simulink model "mod2"  (R2017a)
settings: Solver=VariableStepAuto  StartTime=0.0  StopTime=10.0  RelTol=1e-3
libraries: simulink x2
settings Model: Creator=step_oda  LastModifiedBy=step_oda

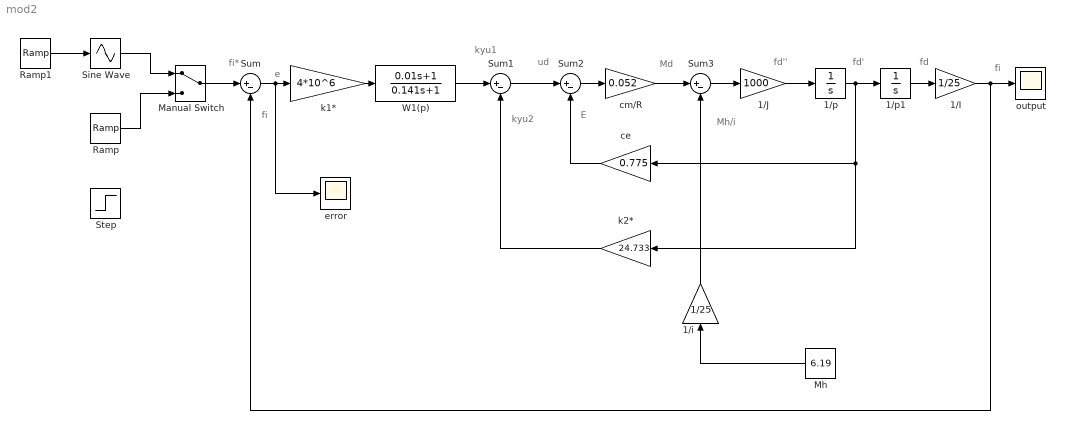
== system mod2 ==
  note: fi
  note: fd
  note: fd'
  note: fd''
  note: ud
  note: Md
  note: fi
  note: e
  note: fi*
  note: kyu1
  note: kyu2
  note: E
  note: Mh/i
  1/I : Gain  Gain=1/25
  1/J : Gain  Gain=1000
  1/i : Gain  Gain=1/25
  1/p : Integrator
  1/p1 : Integrator
  Manual Switch : ManualSwitch
  Mh : Constant  Value=6.19
  Ramp : simulink/Sources/Ramp  slope=4  start=0  X0=0
  Ramp1 : simulink/Sources/Ramp  slope=1  start=0  X0=0
  Sine Wave : Sin  TimeSource=Use external signal  Amplitude=0.533  Frequency=7.5  SampleTime=0
  Step : Step  Time=0  SampleTime=0
  Sum{,1..3} (4 alike) : Sum  Inputs=|+-
  W1(p) : TransferFcn  Numerator=[0.01 1]  Denominator=[0.141 1]
  ce : Gain  Gain=0.775
  cm/R : Gain  Gain=0.052
  "error " : Scope
  k1* : Gain  Gain=4*10^6
  k2* : Gain  Gain=24.733
  output : Scope
  wires:
  1/p1/1 -> 1/I/1
  Manual Switch/1 -> Sum/1
  Sum/1 -> "error "/1, k1*/1
  k1*/1 -> W1(p)/1
  W1(p)/1 -> Sum1/1
  Sum1/1 -> Sum2/1
  Sum2/1 -> cm/R/1
  cm/R/1 -> Sum3/1
  Sum3/1 -> 1/J/1
  1/J/1 -> 1/p/1
  1/p/1 -> k2*/1, ce/1, 1/p1/1
  ce/1 -> Sum2/2
  k2*/1 -> Sum1/2
  1/i/1 -> Sum3/2
  Mh/1 -> 1/i/1
  1/I/1 -> Sum/2, output/1
  Sine Wave/1 -> Manual Switch/1
  Ramp1/1 -> Sine Wave/1
  Ramp/1 -> Manual Switch/2
